simulink model "TCMSSystem"  (R2019b)
settings: configuration reference "ConfigSet_TCMSSystem_Reference" (kept outside this file)
model workspace (MAT data in the model file):
  Prm_TCMSSystem : Simulink.Parameter (value not decoded)
  SampleTime = 0.05
symbols that are objects in the model workspace (value not decoded): Prm_TCMSSystem
undefined symbols (not defined in the file): ADDIntervention, AK1Status, AK2Status, AKContactorStatus, AllDoorsClosed, AllLeftDoorsClosed, AllRightDoorsClosed, APS1Fault, APS1Isolated, APS1OutputVoltage, APS1Status, APS2Fault, APS2Isolated, APS2OutputVoltage, APS2Status, APSKAKContactor, ASCOEnd1, ASCOEnd2, ATBMode, ATCBypassMode, ATCStatusNotOK, ATOMode, ATPLowSpeedCutoutStatus, ATPMode, AuxCompressor, BatteryCurrent, BatteryIsolationContactor, BatteryTemperature, BatteryVoltage, BCG1Fault, BCG1Isolated, BCG1IsolationFailed, BCG1OutputCurrent, BCG1Status, BCG2Fault, BCG2Isolated, BCG2OutputCurrent, BCG2Status, BCGOutputVoltage, BECU1AxleLockedWheelSet1, BECU2AxleLockedWheelSet2, BECUFaulty, BECUMajorFault, BECUMinorFault, BECUStatus, BIC1Inside, BIC1Outside, BIC2Inside, BIC2Outside, Bogie, Bogie1WSPStatus, Bogie2WSPStatus, BogieFaulty, BogieIsolationStatus, BogieSupportedMass, BrakeCylinderPressureGauge, BrakeLoopCBTripped, BrakeLoopOpenTL, BrakeTrainLineStatus, BrakingDemand ... (+215)
libraries: TimersLib x257, simulink x137, LatchesLib x42, VectorOperationsLib x15, TestBenchLib x12, MathOperationsLib x2, FiltersLib x1
(part 5 of 16)

== system TCMSSystem/TCMSSystemPerVehicle/EnabledTCMSVehicle/TCMSDoors/DoorsDisplay/CabTrainDisplay ==
  TCMSConfig : Inport
  ElectricalSignals : Inport  Port=2
  AND : Logic  AllPortsSameDT=off  OutDataTypeStr=boolean
  Bus Selector : BusSelector  OutputSignals=CabActive
  Bus Selector1 : BusSelector  OutputSignals=HasCab
  CabActiveTrainDisplay : Subsystem  TreatAsAtomicUnit=on
  CabInactiveNoDisplay : Subsystem  TreatAsAtomicUnit=on
  Data Type Conversion : DataTypeConversion  OutDataTypeStr=uint32
  If : If
  Merge : Merge
  CabTrainDisplay : Outport
  wires:
  Merge/1 -> CabTrainDisplay/1
  CabInactiveNoDisplay/1(Out1) -> Merge/2
  CabActiveTrainDisplay/1(Out1) -> Merge/1
  If/2 -> CabInactiveNoDisplay/Action
  If/1 -> CabActiveTrainDisplay/Action
  Data Type Conversion/1 -> If/1
  AND/1 -> Data Type Conversion/1
  Bus Selector/1 -> AND/2  "<CabActive>"
  Bus Selector1/1 -> AND/1  "<HasCab>"
  TCMSConfig/1 -> Bus Selector1/1
  ElectricalSignals/1 -> Bus Selector/1, CabActiveTrainDisplay/1(ElectricalSignals)

== system TCMSSystem/TCMSSystemPerVehicle/EnabledTCMSVehicle/TCMSDoors/DoorsDisplay/TCMSVehicleInfo ==
  In Bus Element3 : Inport  PortName=DoorSystem  Element=Doors
  CommonVehicleConfig : Inport  Port=2
  In Bus Element : Inport  Port=3  PortName=ElectricalSignals  Element=DCUPower
  In Bus Element2 : Inport  Port=4  PortName=InputControlStates
  DoorsStatus1 : Subsystem
  OR : Logic  Operator=OR  Inputs=1  AllPortsSameDT=off  OutDataTypeStr=boolean
  Subsystem1 : Subsystem
  TCMSVehicleInfo : Outport
  UnexpectedDoorOpened : Outport  Port=2
  wires:
  In Bus Element3/1 -> DoorsStatus1/1(Doors)  "Doors"
  Subsystem1/1(TCMSDoorStatus) -> TCMSVehicleInfo/1
  CommonVehicleConfig/1 -> Subsystem1/1(CommonVehicleConfig)
  DoorsStatus1/1(DoorOpenStatus) -> Subsystem1/2(DoorOpenStatus)
  DoorsStatus1/16(DLSLFailure) -> Subsystem1/17(DLSLFailure)
  DoorsStatus1/17(DoorMajorFault) -> Subsystem1/18(DoorMajorFault)
  DoorsStatus1/12(DCUFailure) -> Subsystem1/13(DCUFailure)
  DoorsStatus1/3(DoorIsolatedStatus) -> Subsystem1/4(DoorIsolatedStatus)
  DoorsStatus1/15(DLSRFailure) -> Subsystem1/16(DLSRFailure)
  DoorsStatus1/13(DCSRFailure) -> Subsystem1/14(DCSRFailure)
  DoorsStatus1/14(DCSLFailure) -> Subsystem1/15(DCSLFailure)
  DoorsStatus1/10(DoorFailedToUnlock) -> Subsystem1/11(DoorFailedToUnlock)
  DoorsStatus1/4(DoorFaultStatus) -> Subsystem1/5(DoorFaultStatus)
  DoorsStatus1/7(DoorOpenObstruction) -> Subsystem1/8(DoorOpenObstruction)
  DoorsStatus1/8(DoorMotorCircuitFailure) -> Subsystem1/9(DoorMotorCircuitFailure)
  DoorsStatus1/2(DoorEmergencyReleasedStatus) -> Subsystem1/3(DoorEmergencyReleasedStatus)
  DoorsStatus1/6(DoorCloseObstruction) -> Subsystem1/7(DoorCloseObstruction)
  DoorsStatus1/5(DoorLockedStatus) -> Subsystem1/6(DoorLockedStatus)
  DoorsStatus1/11(DoorUnexpectedUnlocking) -> Subsystem1/12(DoorUnexpectedUnlocking)
  DoorsStatus1/9(DoorFailedToLock) -> Subsystem1/10(DoorFailedToLock)
  DoorsStatus1/18(UnexpectedDoorOpeningDetectedByCC) -> OR/1, Subsystem1/19(UnexpectedDoorOpeningDetectedByCC)
  OR/1 -> UnexpectedDoorOpened/1
  In Bus Element/1 -> Subsystem1/20(DCUPower)
  In Bus Element2/1 -> Subsystem1/21(InputControlStates)

== system TCMSSystem/TCMSSystemPerVehicle/EnabledTCMSVehicle/TCMSElectrical/ElectricalControl/Automatic Start Mode ==
  Key_Switch : Inport
  MS : Inport  Port=2
  TBC : Inport  Port=3
  WakeUp : Inport  Port=4
  Compare To Constant : simulink/Logic and Bit Operations/Compare To Constant  relop===  const=0  OutDataTypeStr=boolean
  Compare To Constant1 : simulink/Logic and Bit Operations/Compare To Constant  relop===  const=0  OutDataTypeStr=boolean
  Compare To Constant2 : simulink/Logic and Bit Operations/Compare To Constant  relop===  const=-100  OutDataTypeStr=boolean
  Logical Operator : Logic  Inputs=4  AllPortsSameDT=off  OutDataTypeStr=boolean
  TimerOnDelay NoInit : TimersLib/TimerOnDelay NoInit  UpperSaturationLimit=40  OutputTime=off  SampleTime=-1
      settings: SourceProductName=Sydac Utilities
  AutoStart : Outport
  wires:
  Key_Switch/1 -> Compare To Constant/1
  Compare To Constant/1 -> Logical Operator/1
  MS/1 -> Compare To Constant1/1
  Compare To Constant1/1 -> Logical Operator/2
  TBC/1 -> Compare To Constant2/1
  Compare To Constant2/1 -> Logical Operator/3
  WakeUp/1 -> TimerOnDelay NoInit/1
  Logical Operator/1 -> AutoStart/1
  TimerOnDelay NoInit/1 -> Logical Operator/4

== system TCMSSystem/TCMSSystemPerVehicle/EnabledTCMSVehicle/TCMSElectrical/ElectricalControl/Compressor_Start_Stop ==
  In Bus Element134 : Inport  PortName=PneumaticsSignals  Element=MainReservoirPressureGauge
  ActiveCab : Inport  Port=2
  NonActiveCab : Inport  Port=3
  AND19 : Logic  AllPortsSameDT=off  OutDataTypeStr=boolean
  AND20 : Logic  AllPortsSameDT=off  OutDataTypeStr=boolean
  AND21 : Logic  Operator=OR  AllPortsSameDT=off  OutDataTypeStr=boolean
  Compressor at DM1 : LatchesLib/SR Latch - Reset Priority  initial_condition=0
      settings: SourceProductName=Latches
  Compressor at DM2 : LatchesLib/SR Latch - Reset Priority  initial_condition=0
      settings: SourceProductName=Latches
  Constant3 : Constant  Value=800000
  Constant4 : Constant  Value=750000
  Constant5 : Constant  Value=1000000
  Data Type Conversion : DataTypeConversion
  Relational Operator : RelationalOperator  Operator=<=  OutDataTypeStr=boolean  RndMeth=Simplest
  Relational Operator1 : RelationalOperator  Operator=<=  OutDataTypeStr=boolean  RndMeth=Simplest
  Relational Operator2 : RelationalOperator  OutDataTypeStr=boolean  RndMeth=Simplest
  CompressorCmd : Outport
  wires:
  Relational Operator2/1 -> Compressor at DM2/2, Compressor at DM1/2
  Relational Operator/1 -> AND19/1
  Relational Operator1/1 -> AND20/1
  In Bus Element134/1 -> Relational Operator/1, Relational Operator1/1, Relational Operator2/1
  AND21/1 -> Data Type Conversion/1
  ActiveCab/1 -> AND19/2
  Compressor at DM1/1 -> AND21/1
  Constant4/1 -> Relational Operator1/2
  Compressor at DM2/1 -> AND21/2
  NonActiveCab/1 -> AND20/2
  Constant5/1 -> Relational Operator2/2
  AND19/1 -> Compressor at DM1/1
  AND20/1 -> Compressor at DM2/1
  Constant3/1 -> Relational Operator/2
  Data Type Conversion/1 -> CompressorCmd/1

== system TCMSSystem/TCMSSystemPerVehicle/EnabledTCMSVehicle/TCMSElectrical/ElectricalControl/Doors ==
  BusIn : Inport
  AllLeftDoorsClosed : Inport  Port=2
  Unused : Inport  Port=3
  AllRightDoorsClosed : Inport  Port=4
  AutoMode : Inport  Port=5
  In Bus Element : Inport  Port=6  PortName=ElectricalSignals  Element=LeftDoorEnable
  In Bus Element1 : Inport  Port=6  PortName=ElectricalSignals  Element=RightDoorEnable
  In Bus Element4 : Inport  Port=6  PortName=ElectricalSignals  Element=LeftHoldDoorClose
  In Bus Element5 : Inport  Port=6  PortName=ElectricalSignals  Element=RightHoldDoorClose
  In Bus Element2 : Inport  Port=7  PortName=CBTC  Element=LeftDoorCloseIndicator
  In Bus Element3 : Inport  Port=7  PortName=CBTC  Element=RightDoorCloseIndicator
  Bus Assignment3 : BusAssignment  AssignedSignals=LeftDoorAuth_Closed,LeftDoorAuth_Opened,RightDoorAuth_Closed,RightDoorAuth_Opened,RightDoorAuth_Opened_Op2_5,LeftDoorAuth_Opened_Op2_5,LeftDoorAuth_OpenedOP1,RightDoorAuth_OpenedOP1
  Constant : Constant  Value=0
  Constant1 : Constant  Value=0
  Data Type Conversion{3,12,17..18} (4 alike) : DataTypeConversion
  Demux4 : Demux  Outputs=16
  Mux7 : Mux  Inputs=8
  Mux8 : Mux  Inputs=8
  OR5 : Logic  Inputs=1  AllPortsSameDT=off  OutDataTypeStr=boolean
  OR6 : Logic  Inputs=1  AllPortsSameDT=off  OutDataTypeStr=boolean
  Subsystem4 : Subsystem
  Subsystem5 : Subsystem
  Subsystem6 : Subsystem
  Switch{,1..3} (4 alike) : Switch  Criteria=u2 > Threshold
  Terminator : Terminator
  Terminator1 : Terminator
  BusOut : Outport
  wires:
  Switch/1 -> Bus Assignment3/6
  Switch1/1 -> Bus Assignment3/7
  Data Type Conversion17/1 -> Bus Assignment3/4
  Subsystem6/1(RightDoorsAuth&Closed) -> Data Type Conversion17/1
  Data Type Conversion3/1 -> Bus Assignment3/2
  Data Type Conversion18/1 -> Bus Assignment3/5, [RDAO]
  Data Type Conversion12/1 -> Bus Assignment3/3, [LDAO]
  Bus Assignment3/1 -> BusOut/1
  Subsystem6/2(RightDoorsAuth&Opened) -> Data Type Conversion18/1
  Mux7/1 -> OR5/1
  OR5/1 -> Terminator/1  "LeftDoorsAuthorized"
  [RDAO] -> Switch3/1, Switch/3
  BusIn/1 -> Bus Assignment3/1
  Constant/1 -> Switch/1, Switch1/1
  Mux8/1 -> OR6/1
  Subsystem4/1(LeftDoorsAuth&Closed) -> Data Type Conversion3/1
  Subsystem4/2(LeftDoorsAuth&Opened) -> Data Type Conversion12/1
  Subsystem5/1(DoorAuthorized) -> Demux4/1
  [LDAO] -> Switch2/1, Switch1/3
  AllRightDoorsClosed/1 -> Subsystem6/2(AllRightDoorsClosed)
  OR6/1 -> Terminator1/1  "RightDoorsAuthorized"
  Unused/1 -> Subsystem5/1(In1)
  AllLeftDoorsClosed/1 -> Subsystem4/2(AllLeftDoorsClosed)
  Demux4/9 -> Mux8/1
  Demux4/10 -> Mux8/2
  Demux4/11 -> Mux8/3
  Demux4/12 -> Mux8/4
  Demux4/13 -> Mux8/5
  Demux4/14 -> Mux8/6
  Demux4/15 -> Mux8/7
  Demux4/16 -> Mux8/8
  Demux4/1 -> Mux7/1
  Demux4/2 -> Mux7/2
  Demux4/3 -> Mux7/3
  Demux4/4 -> Mux7/4
  Demux4/5 -> Mux7/5
  Demux4/6 -> Mux7/6
  Demux4/7 -> Mux7/7
  Demux4/8 -> Mux7/8
  In Bus Element/1 -> Subsystem4/1(LeftDoorsEnable)
  In Bus Element1/1 -> Subsystem6/1(RightDoorsEnable)
  In Bus Element2/1 -> Subsystem4/3(ATCLeftDoorCloseAuth)
  In Bus Element3/1 -> Subsystem6/3(ATCRightDoorCloseAuth)
  In Bus Element5/1 -> Subsystem6/4(RightHoldDooorClose)
  In Bus Element4/1 -> Subsystem4/4(LeftHoldDooorClose)
  Constant1/1 -> Switch2/3, Switch3/3
  AutoMode/1 -> Switch/2, Switch3/2, Switch2/2, Switch1/2
  Switch2/1 -> Bus Assignment3/8
  Switch3/1 -> Bus Assignment3/9

== system TCMSSystem/TCMSSystemPerVehicle/EnabledTCMSVehicle/TCMSElectrical/ElectricalControl/Subsystem ==
  note: SH: VCBs are closed by pressing the VCBCPB, hence implemented in electrical system.
      | If there is any new requirement for TCMS to close the VCB (apart from at the end of neutral section) shall be implemented here.
  note: VCB Open command in Faults
  In Bus Element : Inport  PortName=WireStates  Element=TW_POFFPB
  In Bus Element12 : Inport  PortName=WireStates  Element=TW_TPOR
  In Bus Element7 : Inport  Port=2  PortName=Environment  Element=NeutralSection
  In Bus Element1 : Inport  Port=2  PortName=Environment  Element=DamagedOHE
  In Bus Element9 : Inport  Port=2  PortName=Environment  Element=VehiclesPassedNS
  Fault : Inport  Port=3
  In Bus Element2 : Inport  Port=4  PortName=PantographSystem  Element=PantographPosition
  In Bus Element5 : Inport  Port=5  PortName=DisplayControl  Element=TCMSVCBOpenReq
  In Bus Element6 : Inport  Port=5  PortName=DisplayControl  Element=TCMSVCBCloseReq
  In Bus Element3 : Inport  Port=5  PortName=DisplayControl  Element=TCMSVCBResetReq
  In Bus Element8 : Inport  Port=5  PortName=DisplayControl  Element=TCMSReqCtrlVCBNS
  In Bus Element10 : Inport  Port=6  PortName=VCBState
  AND : Logic  AllPortsSameDT=off  OutDataTypeStr=boolean
  AND1 : Logic  AllPortsSameDT=off  OutDataTypeStr=boolean
  Chart : Stateflow chart  BlockKeywords=__PRM__SERIALIZED__DATA__:Stateflow Chart,Stateflow Diagram  TreatAsAtomicUnit=on
  Compare To Constant : simulink/Logic and Bit Operations/Compare To Constant  relop=>=  const=1  OutDataTypeStr=boolean
  Compare To Constant1 : simulink/Logic and Bit Operations/Compare To Constant  relop===  const=1  OutDataTypeStr=boolean
  Data Type Conversion : DataTypeConversion
  Logical Operator1 : Logic  Operator=OR  AllPortsSameDT=off  OutDataTypeStr=boolean
  Logical Operator2 : Logic  Operator=OR  Inputs=3  AllPortsSameDT=off  OutDataTypeStr=boolean
  Logical Operator3 : Logic  AllPortsSameDT=off  OutDataTypeStr=boolean
  Logical Operator4 : Logic  Operator=OR  AllPortsSameDT=off  OutDataTypeStr=boolean
  Logical Operator6 : Logic  Operator=OR  AllPortsSameDT=off  OutDataTypeStr=boolean
  MinimumDurationTimer : TimersLib/MinimumDurationTimer  UpperSaturationLimit=2  SampleTime=-1
      settings: SourceProductName=Sydac Utilities
  NOT : Logic  Operator=NOT  AllPortsSameDT=off  OutDataTypeStr=boolean
  Relational Operator : RelationalOperator  Operator=<  OutDataTypeStr=boolean  RndMeth=Simplest
  Unit Delay : UnitDelay  SampleTime=-1  HasFrameUpgradeWarning=on
  VCBC : Outport
  VCBO : Outport  Port=2
  BackupModeActive : Outport  Port=3
  TrainInNeutralSection : Outport  Port=4
  wires:
  Relational Operator/1 -> MinimumDurationTimer/1
  Logical Operator6/1 -> VCBO/1
  In Bus Element5/1 -> Logical Operator6/2
  Fault/1 -> Logical Operator3/2
  Compare To Constant/1 -> Data Type Conversion/1, Logical Operator3/1
  AND1/1 -> Logical Operator4/1, Unit Delay/1, Relational Operator/1
  In Bus Element1/1 -> Logical Operator4/2
  Logical Operator4/1 -> Logical Operator6/1
  Logical Operator1/1 -> VCBC/1
  MinimumDurationTimer/1 -> Logical Operator1/2
  Unit Delay/1 -> Relational Operator/2
  In Bus Element2/1 -> Compare To Constant1/1
  Compare To Constant1/1 -> Chart/4(PantographRaisedFully), AND/2  "PantographRaisedFully"
  AND/1 -> Logical Operator1/1
  In Bus Element6/1 -> Logical Operator2/2
  Logical Operator2/1 -> AND/1
  In Bus Element3/1 -> Logical Operator2/3
  NOT/1 -> AND1/2
  In Bus Element8/1 -> NOT/1
  In Bus Element7/1 -> AND1/1
  In Bus Element9/1 -> Compare To Constant/1
  Logical Operator3/1 -> BackupModeActive/1
  Data Type Conversion/1 -> TrainInNeutralSection/1
  In Bus Element12/1 -> Chart/1(TW_TPOR)
  Chart/1(VCBCloseReq) -> Logical Operator2/1
  In Bus Element/1 -> Chart/2(TW_POFF)
  In Bus Element10/1 -> Chart/3(VCBState)

== system TCMSSystem/TCMSSystemPerVehicle/EnabledTCMSVehicle/TCMSElectrical/ElectricalControl/Subsystem1 ==
  NonActiveCab : Inport
  HasCab : Inport  Port=2
  Mode : Inport  Port=3
  ActiveCab : Inport  Port=4
  TW_ReverseDirection : Inport  Port=5
  AND1 : Logic  Operator=OR  AllPortsSameDT=off  OutDataTypeStr=boolean
  AND{2,5..6,9} (4 alike) : Logic  AllPortsSameDT=off  OutDataTypeStr=boolean
  AND3 : Logic  Inputs=3  AllPortsSameDT=off  OutDataTypeStr=boolean
  ATO : simulink/Logic and Bit Operations/Compare To Constant  relop===  const=6  OutDataTypeStr=boolean
  ATP : simulink/Logic and Bit Operations/Compare To Constant  relop===  const=1  OutDataTypeStr=boolean
  NotInOFF : simulink/Logic and Bit Operations/Compare To Constant  relop=~=  const=0  OutDataTypeStr=boolean
  NotInStandby : simulink/Logic and Bit Operations/Compare To Constant  relop=~=  const=2  OutDataTypeStr=boolean
  RMF : simulink/Logic and Bit Operations/Compare To Constant  relop===  const=4  OutDataTypeStr=boolean
  RMR : simulink/Logic and Bit Operations/Compare To Constant  relop===  const=3  OutDataTypeStr=boolean
  Switch2 : Switch  Criteria=u2 > Threshold
  XOR : Logic  Operator=XOR  AllPortsSameDT=off  OutDataTypeStr=boolean
  ATPMode : Outport
  DrivingDirection : Outport  Port=2
  RMMode : Outport  Port=3
  AutoMode : Outport  Port=4
  wires:
  Mode/1 -> ATP/1, NotInOFF/1, NotInStandby/1, ATO/1, RMF/1, RMR/1
  HasCab/1 -> AND9/2, AND2/1
  XOR/1 -> RMMode/1  "RM"
  Switch2/1 -> DrivingDirection/1
  ActiveCab/1 -> AND3/2, AND6/2, AND5/2  "ActiveCabForward"
  AND5/1 -> XOR/1
  NonActiveCab/1 -> Switch2/1  "LastCabForward"
  RMF/1 -> AND6/1
  AND6/1 -> XOR/2
  ATP/1 -> AND9/1, AND1/1
  RMR/1 -> AND5/1
  AND9/1 -> ATPMode/1
  ATO/1 -> AND1/2
  AND2/1 -> AutoMode/1
  AND1/1 -> AND2/2
  TW_ReverseDirection/1 -> Switch2/2
  NotInOFF/1 -> AND3/1
  NotInStandby/1 -> AND3/3
  AND3/1 -> Switch2/3  "ActiveCabForward"

== system TCMSSystem/TCMSSystemPerVehicle/EnabledTCMSVehicle/TCMSElectrical/ElectricalControl/Subsystem10 ==
  Fault : Inport
  Cond : Inport  Port=2
  HasVCB : Inport  Port=3
  Reset : Inport  Port=4
  Data Type Conversion : DataTypeConversion
  Logical Operator1 : Logic  Inputs=3  AllPortsSameDT=off  OutDataTypeStr=boolean
  SR Latch - Reset Priority : LatchesLib/SR Latch - Reset Priority  initial_condition=0
      settings: SourceProductName=Latches
  Trig : Outport
  wires:
  Data Type Conversion/1 -> Trig/1
  SR Latch - Reset Priority/1 -> Data Type Conversion/1
  Logical Operator1/1 -> SR Latch - Reset Priority/1
  Fault/1 -> Logical Operator1/1
  Cond/1 -> Logical Operator1/2
  Reset/1 -> SR Latch - Reset Priority/2
  HasVCB/1 -> Logical Operator1/3

== system TCMSSystem/TCMSSystemPerVehicle/EnabledTCMSVehicle/TCMSElectrical/ElectricalControl/Subsystem11 ==
  Fault : Inport
  Cond : Inport  Port=2
  Cond1 : Inport  Port=3
  Data Type Conversion : DataTypeConversion
  Detect Decrease : simulink/Logic and Bit Operations/Detect Decrease  vinit=0.0  OutDataTypeStr=boolean
  Logical Operator1 : Logic  AllPortsSameDT=off  OutDataTypeStr=boolean
  Logical Operator2 : Logic  Operator=OR  AllPortsSameDT=off  OutDataTypeStr=boolean
  SR Latch - Reset Priority : LatchesLib/SR Latch - Reset Priority  initial_condition=0
      settings: SourceProductName=Latches
  Trig : Outport
  wires:
  Data Type Conversion/1 -> Trig/1
  Detect Decrease/1 -> Logical Operator2/1
  SR Latch - Reset Priority/1 -> Data Type Conversion/1
  Logical Operator1/1 -> SR Latch - Reset Priority/1
  Fault/1 -> Logical Operator1/1, Detect Decrease/1
  Cond/1 -> Logical Operator1/2
  Logical Operator2/1 -> SR Latch - Reset Priority/2
  Cond1/1 -> Logical Operator2/2

== system TCMSSystem/TCMSSystemPerVehicle/EnabledTCMSVehicle/TCMSElectrical/ElectricalControl/Subsystem12 ==
  Fault : Inport
  Cond : Inport  Port=2
  Cond1 : Inport  Port=3
  Data Type Conversion : DataTypeConversion
  Detect Decrease : simulink/Logic and Bit Operations/Detect Decrease  vinit=0.0  OutDataTypeStr=boolean
  Logical Operator1 : Logic  AllPortsSameDT=off  OutDataTypeStr=boolean
  Logical Operator2 : Logic  Operator=OR  AllPortsSameDT=off  OutDataTypeStr=boolean
  SR Latch - Reset Priority : LatchesLib/SR Latch - Reset Priority  initial_condition=0
      settings: SourceProductName=Latches
  Trig : Outport
  wires:
  Cond/1 -> Logical Operator1/2
  Fault/1 -> Detect Decrease/1, Logical Operator1/1
  Logical Operator1/1 -> SR Latch - Reset Priority/1
  SR Latch - Reset Priority/1 -> Data Type Conversion/1
  Detect Decrease/1 -> Logical Operator2/1
  Data Type Conversion/1 -> Trig/1
  Logical Operator2/1 -> SR Latch - Reset Priority/2
  Cond1/1 -> Logical Operator2/2

== system TCMSSystem/TCMSSystemPerVehicle/EnabledTCMSVehicle/TCMSElectrical/ElectricalControl/Subsystem13 ==
  Fault : Inport
  Cond : Inport  Port=2
  Cond1 : Inport  Port=3
  Data Type Conversion : DataTypeConversion
  Detect Decrease : simulink/Logic and Bit Operations/Detect Decrease  vinit=0.0  OutDataTypeStr=boolean
  Logical Operator1 : Logic  AllPortsSameDT=off  OutDataTypeStr=boolean
  Logical Operator2 : Logic  Operator=OR  AllPortsSameDT=off  OutDataTypeStr=boolean
  SR Latch - Reset Priority : LatchesLib/SR Latch - Reset Priority  initial_condition=0
      settings: SourceProductName=Latches
  Trig : Outport
  wires:
  Cond/1 -> Logical Operator1/2
  Fault/1 -> Detect Decrease/1, Logical Operator1/1
  Logical Operator1/1 -> SR Latch - Reset Priority/1
  SR Latch - Reset Priority/1 -> Data Type Conversion/1
  Detect Decrease/1 -> Logical Operator2/1
  Data Type Conversion/1 -> Trig/1
  Cond1/1 -> Logical Operator2/2
  Logical Operator2/1 -> SR Latch - Reset Priority/2

== system TCMSSystem/TCMSSystemPerVehicle/EnabledTCMSVehicle/TCMSElectrical/ElectricalControl/Subsystem14 ==
  Fault : Inport
  Cond : Inport  Port=2
  Cond1 : Inport  Port=3
  Data Type Conversion : DataTypeConversion
  Detect Decrease : simulink/Logic and Bit Operations/Detect Decrease  vinit=0.0  OutDataTypeStr=boolean
  Logical Operator1 : Logic  AllPortsSameDT=off  OutDataTypeStr=boolean
  Logical Operator2 : Logic  Operator=OR  AllPortsSameDT=off  OutDataTypeStr=boolean
  SR Latch - Reset Priority : LatchesLib/SR Latch - Reset Priority  initial_condition=0
      settings: SourceProductName=Latches
  Trig : Outport
  wires:
  Data Type Conversion/1 -> Trig/1
  Detect Decrease/1 -> Logical Operator2/1
  SR Latch - Reset Priority/1 -> Data Type Conversion/1
  Logical Operator1/1 -> SR Latch - Reset Priority/1
  Fault/1 -> Logical Operator1/1, Detect Decrease/1
  Cond/1 -> Logical Operator1/2
  Cond1/1 -> Logical Operator2/2
  Logical Operator2/1 -> SR Latch - Reset Priority/2

== system TCMSSystem/TCMSSystemPerVehicle/EnabledTCMSVehicle/TCMSElectrical/ElectricalControl/Subsystem15 ==
  Fault : Inport
  Cond : Inport  Port=2
  Data Type Conversion : DataTypeConversion
  Detect Decrease : simulink/Logic and Bit Operations/Detect Decrease  vinit=0.0  OutDataTypeStr=boolean
  Logical Operator1 : Logic  AllPortsSameDT=off  OutDataTypeStr=boolean
  SR Latch - Reset Priority : LatchesLib/SR Latch - Reset Priority  initial_condition=0
      settings: SourceProductName=Latches
  Trig : Outport
  wires:
  Cond/1 -> Logical Operator1/2
  Fault/1 -> Detect Decrease/1, Logical Operator1/1
  Logical Operator1/1 -> SR Latch - Reset Priority/1
  SR Latch - Reset Priority/1 -> Data Type Conversion/1
  Detect Decrease/1 -> SR Latch - Reset Priority/2
  Data Type Conversion/1 -> Trig/1

== system TCMSSystem/TCMSSystemPerVehicle/EnabledTCMSVehicle/TCMSElectrical/ElectricalControl/Subsystem16 ==
  Fault : Inport
  Cond : Inport  Port=2
  Data Type Conversion : DataTypeConversion
  Detect Decrease : simulink/Logic and Bit Operations/Detect Decrease  vinit=0.0  OutDataTypeStr=boolean
  Logical Operator1 : Logic  AllPortsSameDT=off  OutDataTypeStr=boolean
  SR Latch - Reset Priority : LatchesLib/SR Latch - Reset Priority  initial_condition=0
      settings: SourceProductName=Latches
  Trig : Outport
  wires:
  Data Type Conversion/1 -> Trig/1
  Detect Decrease/1 -> SR Latch - Reset Priority/2
  SR Latch - Reset Priority/1 -> Data Type Conversion/1
  Logical Operator1/1 -> SR Latch - Reset Priority/1
  Fault/1 -> Logical Operator1/1, Detect Decrease/1
  Cond/1 -> Logical Operator1/2

== system TCMSSystem/TCMSSystemPerVehicle/EnabledTCMSVehicle/TCMSElectrical/ElectricalControl/Subsystem17 ==
  Fault : Inport
  Cond : Inport  Port=2
  Cond1 : Inport  Port=3
  Data Type Conversion : DataTypeConversion
  Detect Decrease : simulink/Logic and Bit Operations/Detect Decrease  vinit=0.0  OutDataTypeStr=boolean
  Logical Operator1 : Logic  AllPortsSameDT=off  OutDataTypeStr=boolean
  Logical Operator2 : Logic  Operator=OR  AllPortsSameDT=off  OutDataTypeStr=boolean
  SR Latch - Reset Priority : LatchesLib/SR Latch - Reset Priority  initial_condition=0
      settings: SourceProductName=Latches
  Trig : Outport
  wires:
  Cond/1 -> Logical Operator1/2
  Fault/1 -> Detect Decrease/1, Logical Operator1/1
  Logical Operator1/1 -> SR Latch - Reset Priority/1
  SR Latch - Reset Priority/1 -> Data Type Conversion/1
  Detect Decrease/1 -> Logical Operator2/1
  Data Type Conversion/1 -> Trig/1
  Logical Operator2/1 -> SR Latch - Reset Priority/2
  Cond1/1 -> Logical Operator2/2

== system TCMSSystem/TCMSSystemPerVehicle/EnabledTCMSVehicle/TCMSElectrical/ElectricalControl/Subsystem18 ==
  Fault : Inport
  Cond : Inport  Port=2
  Cond1 : Inport  Port=3
  Data Type Conversion : DataTypeConversion
  Detect Decrease : simulink/Logic and Bit Operations/Detect Decrease  vinit=0.0  OutDataTypeStr=boolean
  Logical Operator1 : Logic  AllPortsSameDT=off  OutDataTypeStr=boolean
  Logical Operator2 : Logic  Operator=OR  AllPortsSameDT=off  OutDataTypeStr=boolean
  SR Latch - Reset Priority : LatchesLib/SR Latch - Reset Priority  initial_condition=0
      settings: SourceProductName=Latches
  Trig : Outport
  wires:
  Data Type Conversion/1 -> Trig/1
  Detect Decrease/1 -> Logical Operator2/1
  SR Latch - Reset Priority/1 -> Data Type Conversion/1
  Logical Operator1/1 -> SR Latch - Reset Priority/1
  Fault/1 -> Logical Operator1/1, Detect Decrease/1
  Cond/1 -> Logical Operator1/2
  Cond1/1 -> Logical Operator2/2
  Logical Operator2/1 -> SR Latch - Reset Priority/2

== system TCMSSystem/TCMSSystemPerVehicle/EnabledTCMSVehicle/TCMSElectrical/ElectricalControl/Subsystem19 ==
  Open : Inport
  Close : Inport  Port=2
  Data Type Conversion : DataTypeConversion
  Logical Operator1 : Logic  AllPortsSameDT=off  OutDataTypeStr=boolean
  Logical Operator2 : Logic  Operator=NOT  AllPortsSameDT=off  OutDataTypeStr=boolean
  Trig : Outport
  wires:
  Open/1 -> Logical Operator1/1
  Close/1 -> Logical Operator2/1
  Logical Operator1/1 -> Data Type Conversion/1
  Logical Operator2/1 -> Logical Operator1/2
  Data Type Conversion/1 -> Trig/1

== system TCMSSystem/TCMSSystemPerVehicle/EnabledTCMSVehicle/TCMSElectrical/ElectricalControl/Subsystem2 ==
  TW_POFF : Inport
  TSDR_ON : Inport  Port=2
  KeySwitchStatus : Inport  Port=3
  ShutdownFailure : Inport  Port=4
  TW_ShutdownFailure : Inport  Port=5
  Logical Operator : Logic  Inputs=3  AllPortsSameDT=off  OutDataTypeStr=boolean
  Logical Operator1 : Logic  Operator=NOT  AllPortsSameDT=off  OutDataTypeStr=boolean
  Logical Operator2 : Logic  Operator=NOT  AllPortsSameDT=off  OutDataTypeStr=boolean
  Logical Operator3 : Logic  AllPortsSameDT=off  OutDataTypeStr=boolean
  Logical Operator4 : Logic  Operator=NOT  AllPortsSameDT=off  OutDataTypeStr=boolean
  TimerOnDelay NoInit : TimersLib/TimerOnDelay NoInit  UpperSaturationLimit=5  OutputTime=off  SampleTime=-1
      settings: SourceProductName=Sydac Utilities
  TSDDR : Outport
  TCMS_TSDR : Outport  Port=2
  wires:
  TW_POFF/1 -> Logical Operator/1
  TSDR_ON/1 -> Logical Operator3/1
  TimerOnDelay NoInit/1 -> TSDDR/1
  KeySwitchStatus/1 -> Logical Operator1/1
  Logical Operator1/1 -> Logical Operator/2
  Logical Operator/1 -> TCMS_TSDR/1
  ShutdownFailure/1 -> Logical Operator2/1
  Logical Operator2/1 -> Logical Operator/3
  Logical Operator3/1 -> TimerOnDelay NoInit/1
  TW_ShutdownFailure/1 -> Logical Operator4/1
  Logical Operator4/1 -> Logical Operator3/2

== system TCMSSystem/TCMSSystemPerVehicle/EnabledTCMSVehicle/TCMSElectrical/ElectricalControl/Subsystem20 ==
  Open : Inport
  Close : Inport  Port=2
  Data Type Conversion : DataTypeConversion
  Logical Operator1 : Logic  AllPortsSameDT=off  OutDataTypeStr=boolean
  Logical Operator2 : Logic  Operator=NOT  AllPortsSameDT=off  OutDataTypeStr=boolean
  Trig : Outport
  wires:
  Logical Operator2/1 -> Logical Operator1/2
  Logical Operator1/1 -> Data Type Conversion/1
  Close/1 -> Logical Operator2/1
  Open/1 -> Logical Operator1/1
  Data Type Conversion/1 -> Trig/1

== system TCMSSystem/TCMSSystemPerVehicle/EnabledTCMSVehicle/TCMSElectrical/ElectricalControl/Subsystem21 ==
  Open : Inport
  Close : Inport  Port=2
  Data Type Conversion : DataTypeConversion
  Logical Operator1 : Logic  AllPortsSameDT=off  OutDataTypeStr=boolean
  Logical Operator2 : Logic  Operator=NOT  AllPortsSameDT=off  OutDataTypeStr=boolean
  Trig : Outport
  wires:
  Open/1 -> Logical Operator1/1
  Close/1 -> Logical Operator2/1
  Logical Operator1/1 -> Data Type Conversion/1
  Logical Operator2/1 -> Logical Operator1/2
  Data Type Conversion/1 -> Trig/1

== system TCMSSystem/TCMSSystemPerVehicle/EnabledTCMSVehicle/TCMSElectrical/ElectricalControl/Subsystem22 ==
  Open : Inport
  Close : Inport  Port=2
  Data Type Conversion : DataTypeConversion
  Logical Operator1 : Logic  AllPortsSameDT=off  OutDataTypeStr=boolean
  Logical Operator2 : Logic  Operator=NOT  AllPortsSameDT=off  OutDataTypeStr=boolean
  Trig : Outport
  wires:
  Logical Operator2/1 -> Logical Operator1/2
  Logical Operator1/1 -> Data Type Conversion/1
  Close/1 -> Logical Operator2/1
  Open/1 -> Logical Operator1/1
  Data Type Conversion/1 -> Trig/1

== system TCMSSystem/TCMSSystemPerVehicle/EnabledTCMSVehicle/TCMSElectrical/ElectricalControl/Subsystem3 ==
  Fault : Inport
  LV : Inport  Port=2
  Data Type Conversion : DataTypeConversion
  Detect Decrease : simulink/Logic and Bit Operations/Detect Decrease  vinit=0.0  OutDataTypeStr=boolean
  Logical Operator1 : Logic  AllPortsSameDT=off  OutDataTypeStr=boolean
  SR Latch - Reset Priority : LatchesLib/SR Latch - Reset Priority  initial_condition=0
      settings: SourceProductName=Latches
  Trig : Outport
  wires:
  LV/1 -> Logical Operator1/2
  Fault/1 -> Detect Decrease/1, Logical Operator1/1
  Logical Operator1/1 -> SR Latch - Reset Priority/1
  SR Latch - Reset Priority/1 -> Data Type Conversion/1
  Detect Decrease/1 -> SR Latch - Reset Priority/2
  Data Type Conversion/1 -> Trig/1

== system TCMSSystem/TCMSSystemPerVehicle/EnabledTCMSVehicle/TCMSElectrical/ElectricalControl/Subsystem4 ==
  Fault : Inport
  LV : Inport  Port=2
  Data Type Conversion : DataTypeConversion
  Detect Decrease : simulink/Logic and Bit Operations/Detect Decrease  vinit=0.0  OutDataTypeStr=boolean
  Logical Operator1 : Logic  AllPortsSameDT=off  OutDataTypeStr=boolean
  SR Latch - Reset Priority : LatchesLib/SR Latch - Reset Priority  initial_condition=0
      settings: SourceProductName=Latches
  Trig : Outport
  wires:
  Data Type Conversion/1 -> Trig/1
  Detect Decrease/1 -> SR Latch - Reset Priority/2
  SR Latch - Reset Priority/1 -> Data Type Conversion/1
  Logical Operator1/1 -> SR Latch - Reset Priority/1
  Fault/1 -> Logical Operator1/1, Detect Decrease/1
  LV/1 -> Logical Operator1/2

== system TCMSSystem/TCMSSystemPerVehicle/EnabledTCMSVehicle/TCMSElectrical/ElectricalControl/Subsystem5 ==
  Fault : Inport
  VCB : Inport  Port=2
  Data Type Conversion : DataTypeConversion
  Detect Decrease : simulink/Logic and Bit Operations/Detect Decrease  vinit=0.0  OutDataTypeStr=boolean
  Logical Operator1 : Logic  AllPortsSameDT=off  OutDataTypeStr=boolean
  SR Latch - Reset Priority : LatchesLib/SR Latch - Reset Priority  initial_condition=0
      settings: SourceProductName=Latches
  Trig : Outport
  wires:
  VCB/1 -> Logical Operator1/2
  Fault/1 -> Detect Decrease/1, Logical Operator1/1
  Logical Operator1/1 -> SR Latch - Reset Priority/1
  SR Latch - Reset Priority/1 -> Data Type Conversion/1
  Detect Decrease/1 -> SR Latch - Reset Priority/2
  Data Type Conversion/1 -> Trig/1

== system TCMSSystem/TCMSSystemPerVehicle/EnabledTCMSVehicle/TCMSElectrical/ElectricalControl/Subsystem6 ==
  Fault : Inport
  VCB : Inport  Port=2
  Data Type Conversion : DataTypeConversion
  Detect Decrease : simulink/Logic and Bit Operations/Detect Decrease  vinit=0.0  OutDataTypeStr=boolean
  Logical Operator1 : Logic  AllPortsSameDT=off  OutDataTypeStr=boolean
  SR Latch - Reset Priority : LatchesLib/SR Latch - Reset Priority  initial_condition=0
      settings: SourceProductName=Latches
  Trig : Outport
  wires:
  Data Type Conversion/1 -> Trig/1
  Detect Decrease/1 -> SR Latch - Reset Priority/2
  SR Latch - Reset Priority/1 -> Data Type Conversion/1
  Logical Operator1/1 -> SR Latch - Reset Priority/1
  Fault/1 -> Logical Operator1/1, Detect Decrease/1
  VCB/1 -> Logical Operator1/2

== system TCMSSystem/TCMSSystemPerVehicle/EnabledTCMSVehicle/TCMSElectrical/ElectricalControl/Subsystem7 ==
  Fault : Inport
  VCB : Inport  Port=2
  Data Type Conversion : DataTypeConversion
  Detect Decrease : simulink/Logic and Bit Operations/Detect Decrease  vinit=0.0  OutDataTypeStr=boolean
  Logical Operator1 : Logic  AllPortsSameDT=off  OutDataTypeStr=boolean
  SR Latch - Reset Priority : LatchesLib/SR Latch - Reset Priority  initial_condition=0
      settings: SourceProductName=Latches
  Trig : Outport
  wires:
  VCB/1 -> Logical Operator1/2
  Fault/1 -> Detect Decrease/1, Logical Operator1/1
  Logical Operator1/1 -> SR Latch - Reset Priority/1
  SR Latch - Reset Priority/1 -> Data Type Conversion/1
  Detect Decrease/1 -> SR Latch - Reset Priority/2
  Data Type Conversion/1 -> Trig/1

== system TCMSSystem/TCMSSystemPerVehicle/EnabledTCMSVehicle/TCMSElectrical/ElectricalControl/Subsystem8 ==
  Fault : Inport
  VCB : Inport  Port=2
  Data Type Conversion : DataTypeConversion
  Detect Decrease : simulink/Logic and Bit Operations/Detect Decrease  vinit=0.0  OutDataTypeStr=boolean
  Logical Operator1 : Logic  AllPortsSameDT=off  OutDataTypeStr=boolean
  SR Latch - Reset Priority : LatchesLib/SR Latch - Reset Priority  initial_condition=0
      settings: SourceProductName=Latches
  Trig : Outport
  wires:
  Data Type Conversion/1 -> Trig/1
  Detect Decrease/1 -> SR Latch - Reset Priority/2
  SR Latch - Reset Priority/1 -> Data Type Conversion/1
  Logical Operator1/1 -> SR Latch - Reset Priority/1
  Fault/1 -> Logical Operator1/1, Detect Decrease/1
  VCB/1 -> Logical Operator1/2

== system TCMSSystem/TCMSSystemPerVehicle/EnabledTCMSVehicle/TCMSElectrical/ElectricalControl/Subsystem9 ==
  Fault : Inport
  Cond : Inport  Port=2
  Data Type Conversion : DataTypeConversion
  Detect Decrease : simulink/Logic and Bit Operations/Detect Decrease  vinit=0.0  OutDataTypeStr=boolean
  Logical Operator1 : Logic  AllPortsSameDT=off  OutDataTypeStr=boolean
  SR Latch - Reset Priority : LatchesLib/SR Latch - Reset Priority  initial_condition=0
      settings: SourceProductName=Latches
  Trig : Outport
  wires:
  Cond/1 -> Logical Operator1/2
  Fault/1 -> Detect Decrease/1, Logical Operator1/1
  Logical Operator1/1 -> SR Latch - Reset Priority/1
  SR Latch - Reset Priority/1 -> Data Type Conversion/1
  Detect Decrease/1 -> SR Latch - Reset Priority/2
  Data Type Conversion/1 -> Trig/1

== system TCMSSystem/TCMSSystemPerVehicle/EnabledTCMSVehicle/TCMSElectrical/ElectricalDisplay/APSScreen ==
  note: BatteryScreen
  BusIn : Inport
  In Bus Element8 : Inport  Port=2  PortName=ElectricalSignals  Element=APS1Status
  In Bus Element9 : Inport  Port=2  PortName=ElectricalSignals  Element=APS2Status
  In Bus Element27 : Inport  Port=2  PortName=ElectricalSignals  Element=APS1Fault
  In Bus Element28 : Inport  Port=2  PortName=ElectricalSignals  Element=APS2Fault
  In Bus Element29 : Inport  Port=2  PortName=ElectricalSignals  Element=APS1Isolated
  In Bus Element30 : Inport  Port=2  PortName=ElectricalSignals  Element=APS2Isolated
  In Bus Element31 : Inport  Port=2  PortName=ElectricalSignals  Element=APS1OutputVoltage
  In Bus Element32 : Inport  Port=2  PortName=ElectricalSignals  Element=APS2OutputVoltage
  In Bus Element33 : Inport  Port=2  PortName=ElectricalSignals  Element=AK1Status
  In Bus Element34 : Inport  Port=2  PortName=ElectricalSignals  Element=AK2Status
  In Bus Element35 : Inport  Port=2  PortName=ElectricalSignals  Element=K1Status
  In Bus Element36 : Inport  Port=2  PortName=ElectricalSignals  Element=K2Status
  In Bus Element1 : Inport  Port=2  PortName=ElectricalSignals  Element=APSCBTripped
  Bus Assignment2 : BusAssignment  AssignedSignals=APS1Status,APS2Status,AK1Status,K1Status,AK2Status,K2Status,APS1Isolated,APS2Isolated,APS1OutputVoltage,APS2OutputVoltage,APS1Fault,APS2Fault
  Data Type Conversion{2,8..11,21..22,25..27} (10 alike) : DataTypeConversion
  Logical Operator : Logic  Operator=OR  AllPortsSameDT=off  OutDataTypeStr=boolean
  Logical Operator1 : Logic  Operator=OR  AllPortsSameDT=off  OutDataTypeStr=boolean
  BusOut : Outport
  wires:
  In Bus Element32/1 -> Bus Assignment2/11
  In Bus Element31/1 -> Bus Assignment2/10
  Bus Assignment2/1 -> BusOut/1
  Data Type Conversion9/1 -> Bus Assignment2/4
  In Bus Element30/1 -> Data Type Conversion2/1
  Data Type Conversion22/1 -> Bus Assignment2/6
  Data Type Conversion25/1 -> Bus Assignment2/12
  Data Type Conversion8/1 -> Bus Assignment2/5
  Data Type Conversion2/1 -> Bus Assignment2/9
  BusIn/1 -> Bus Assignment2/1
  In Bus Element28/1 -> Logical Operator/1
  Data Type Conversion27/1 -> Bus Assignment2/8
  Data Type Conversion26/1 -> Bus Assignment2/13
  In Bus Element34/1 -> Data Type Conversion22/1
  Data Type Conversion10/1 -> Bus Assignment2/2
  In Bus Element8/1 -> Data Type Conversion10/1
  In Bus Element9/1 -> Data Type Conversion11/1
  In Bus Element29/1 -> Data Type Conversion27/1
  In Bus Element35/1 -> Data Type Conversion8/1
  Data Type Conversion21/1 -> Bus Assignment2/7
  Data Type Conversion11/1 -> Bus Assignment2/3
  In Bus Element33/1 -> Data Type Conversion9/1
  In Bus Element27/1 -> Logical Operator1/1
  In Bus Element36/1 -> Data Type Conversion21/1
  In Bus Element1/1 -> Logical Operator/2, Logical Operator1/2
  Logical Operator1/1 -> Data Type Conversion25/1
  Logical Operator/1 -> Data Type Conversion26/1

== system TCMSSystem/TCMSSystemPerVehicle/EnabledTCMSVehicle/TCMSElectrical/ElectricalDisplay/BatteryScreen ==
  note: BatteryScreen
  BusIn : Inport
  In Bus Element4 : Inport  Port=2  PortName=ElectricalSignals  Element=BCG1Status
  In Bus Element5 : Inport  Port=2  PortName=ElectricalSignals  Element=BCG2Status
  In Bus Element6 : Inport  Port=2  PortName=ElectricalSignals  Element=BCGOutputVoltage
  In Bus Element7 : Inport  Port=2  PortName=ElectricalSignals  Element=BCG1OutputCurrent
  In Bus Element8 : Inport  Port=2  PortName=ElectricalSignals  Element=BCG2OutputCurrent
  In Bus Element : Inport  Port=2  PortName=ElectricalSignals  Element=BatteryVoltage
  In Bus Element1 : Inport  Port=2  PortName=ElectricalSignals  Element=BatteryCurrent
  In Bus Element2 : Inport  Port=2  PortName=ElectricalSignals  Element=BatteryTemperature
  In Bus Element3 : Inport  Port=2  PortName=ElectricalSignals  Element=BCG1Fault
  In Bus Element9 : Inport  Port=2  PortName=ElectricalSignals  Element=BCG2Fault
  In Bus Element11 : Inport  Port=2  PortName=ElectricalSignals  Element=BCG1Isolated
  In Bus Element12 : Inport  Port=2  PortName=ElectricalSignals  Element=BCG2Isolated
  In Bus Element10 : Inport  Port=2  PortName=ElectricalSignals  Element=BCG1IsolationFailed
  Add : Sum
  Bus Assignment2 : BusAssignment  AssignedSignals=BCG1Status,BCG2Status,BCG1Fault,BCG2Fault,BCGOutputVoltage,BCG1OutputCurrent,BCG2OutputCurrent,TotalOutputCurrent,BatteryVoltage,BatteryCurrent,BatteryTemperature,BCG1Isolated,BCG2Isolated,BCG1IsolationFailed
  Data Type Conversion1 : DataTypeConversion
  Data Type Conversion28 : DataTypeConversion
  BusOut : Outport
  wires:
  In Bus Element4/1 -> Data Type Conversion1/1
  Bus Assignment2/1 -> BusOut/1
  BusIn/1 -> Bus Assignment2/1
  In Bus Element5/1 -> Data Type Conversion28/1
  In Bus Element6/1 -> Bus Assignment2/6
  In Bus Element/1 -> Bus Assignment2/10
  In Bus Element1/1 -> Bus Assignment2/11
  In Bus Element2/1 -> Bus Assignment2/12
  Data Type Conversion28/1 -> Bus Assignment2/3
  Data Type Conversion1/1 -> Bus Assignment2/2
  In Bus Element7/1 -> Add/1, Bus Assignment2/7
  Add/1 -> Bus Assignment2/9
  In Bus Element8/1 -> Add/2, Bus Assignment2/8
  In Bus Element3/1 -> Bus Assignment2/4
  In Bus Element9/1 -> Bus Assignment2/5
  In Bus Element11/1 -> Bus Assignment2/13
  In Bus Element12/1 -> Bus Assignment2/14
  In Bus Element10/1 -> Bus Assignment2/15

== system TCMSSystem/TCMSSystemPerVehicle/EnabledTCMSVehicle/TCMSElectrical/ElectricalDisplay/BrakeLoopInterlock ==
  note: BrakeLoopInterlockScreen
  BusIn : Inport
  In Bus Element : Inport  Port=2  PortName=PantographSignals  Element=BrakeLoopADDIntervention
  In Bus Element2 : Inport  Port=3  PortName=ElectricalTrainWire  Element=BrakeLoopCBTripped
  Bus Assignment7 : BusAssignment  AssignedSignals=ADDIntervention,BrakeLoopCBTripped
  Data Type Conversion : DataTypeConversion
  Data Type Conversion1 : DataTypeConversion
  BusOut : Outport
  wires:
  Bus Assignment7/1 -> BusOut/1
  BusIn/1 -> Bus Assignment7/1
  In Bus Element/1 -> Data Type Conversion/1
  Data Type Conversion/1 -> Bus Assignment7/2
  In Bus Element2/1 -> Data Type Conversion1/1
  Data Type Conversion1/1 -> Bus Assignment7/3

== system TCMSSystem/TCMSSystemPerVehicle/EnabledTCMSVehicle/TCMSElectrical/ElectricalDisplay/BrakeScreen ==
  note: BatteryScreen
  BusIn : Inport
  In Bus Element18 : Inport  Port=2  PortName=ElectricalSignals  Element=BrakeTrainLine
  In Bus Element19 : Inport  Port=2  PortName=ElectricalSignals  Element=MotorTrainLine
  In Bus Element20 : Inport  Port=2  PortName=ElectricalSignals  Element=FSB1Line
  In Bus Element21 : Inport  Port=2  PortName=ElectricalSignals  Element=FSB2Line
  In Bus Element22 : Inport  Port=2  PortName=ElectricalSignals  Element=EB1Line
  In Bus Element23 : Inport  Port=2  PortName=ElectricalSignals  Element=EB2Line
  Bus Assignment2 : BusAssignment  AssignedSignals=BrakeTrainLineStatus,MotorTrainLineStatus,FSB1LineStatus,FSB2LineStatus,EB1LineStatus,EB2LineStatus
  Data Type Conversion{13,15..19} (6 alike) : DataTypeConversion
  BusOut : Outport
  wires:
  BusIn/1 -> Bus Assignment2/1
  Bus Assignment2/1 -> BusOut/1
  Data Type Conversion16/1 -> Bus Assignment2/4
  Data Type Conversion13/1 -> Bus Assignment2/2
  In Bus Element23/1 -> Data Type Conversion19/1
  Data Type Conversion18/1 -> Bus Assignment2/6
  In Bus Element19/1 -> Data Type Conversion15/1
  In Bus Element18/1 -> Data Type Conversion13/1
  In Bus Element21/1 -> Data Type Conversion17/1
  Data Type Conversion17/1 -> Bus Assignment2/5
  Data Type Conversion15/1 -> Bus Assignment2/3
  In Bus Element22/1 -> Data Type Conversion18/1
  Data Type Conversion19/1 -> Bus Assignment2/7
  In Bus Element20/1 -> Data Type Conversion16/1

== system TCMSSystem/TCMSSystemPerVehicle/EnabledTCMSVehicle/TCMSElectrical/ElectricalDisplay/EBLoopInterlockScreen ==
  note: EBLoopInterlockScreen
  BusIn : Inport
  In Bus Element : Inport  Port=2  PortName=ElectricalSignals  Element=EBbyNonCabEnabled
  In Bus Element1 : Inport  Port=2  PortName=ElectricalSignals  Element=EBbyMC
  In Bus Element2 : Inport  Port=2  PortName=ElectricalSignals  Element=EBbyBrakeLoop
  In Bus Element3 : Inport  Port=2  PortName=ElectricalSignals  Element=EBbyDeadMan
  In Bus Element4 : Inport  Port=2  PortName=ElectricalSignals  Element=EBApplied
  In Bus Element13 : Inport  Port=2  PortName=ElectricalSignals  Element=EBApplied
  In Bus Element11 : Inport  Port=2  PortName=ElectricalSignals  Element=CabActive
  In Bus Element7 : Inport  Port=2  PortName=ElectricalSignals  Element=CabActive
  In Bus Element8 : Inport  Port=2  PortName=ElectricalSignals  Element=EBbyCC
  In Bus Element9 : Inport  Port=2  PortName=ElectricalSignals  Element=EBdueToATCZeroSpeed
  In Bus Element6 : Inport  Port=2  PortName=ElectricalSignals  Element=EBbyPB
  In Bus Element10 : Inport  Port=2  PortName=ElectricalSignals  Element=ZeroSpeed
  In Bus Element5 : Inport  Port=3  PortName=InputControls  Element=ModeSelector
  In Bus Element12 : Inport  Port=4  PortName=TCMSSystemVehicleConfig  Element=IsFirstVehicle
  AND{1,3,5..8} (6 alike) : Logic  Inputs=3  AllPortsSameDT=off  OutDataTypeStr=boolean
  AND{10,12..14} (4 alike) : Logic  Operator=NOT  AllPortsSameDT=off  OutDataTypeStr=boolean
  AND{2,4,9,11} (4 alike) : Logic  AllPortsSameDT=off  OutDataTypeStr=boolean
  Bus Assignment7 : BusAssignment  AssignedSignals=EBForNonCabEnabled,EBForNonDirectionSelected,EBDueToPushButton,EBByMC,EBByBrakeLoop,EBDueToDeadman,EBByCC,EBDueToATCZeroSpeed
  Data Type Conversion{1..2,40,43..47} (8 alike) : DataTypeConversion
  OFF : simulink/Logic and Bit Operations/Compare To Constant  relop===  const=0  OutDataTypeStr=boolean
  OR : Logic  Operator=OR  AllPortsSameDT=off  OutDataTypeStr=boolean
  SR Latch - Reset Priority : LatchesLib/SR Latch - Reset Priority  initial_condition=0
      settings: SourceProductName=Latches
  SR Latch - Reset Priority1 : LatchesLib/SR Latch - Reset Priority  initial_condition=0
      settings: SourceProductName=Latches
  Standby : simulink/Logic and Bit Operations/Compare To Constant  relop===  const=2  OutDataTypeStr=boolean
  Terminator : Terminator
  BusOut : Outport
  wires:
  In Bus Element4/1 -> AND8/1, AND7/1, AND2/1, AND3/2, AND1/2, AND4/2, AND5/2, AND6/2
  Bus Assignment7/1 -> BusOut/1
  AND3/1 -> Data Type Conversion40/1
  AND1/1 -> Data Type Conversion46/1
  In Bus Element2/1 -> AND5/1
  AND6/1 -> Data Type Conversion45/1
  OFF/1 -> OR/1
  Data Type Conversion40/1 -> Bus Assignment7/2
  AND2/1 -> Data Type Conversion47/1
  In Bus Element5/1 -> OFF/1, Standby/1
  In Bus Element6/1 -> AND2/2
  AND5/1 -> Data Type Conversion44/1
  In Bus Element3/1 -> AND6/1
  In Bus Element1/1 -> AND4/1
  Standby/1 -> OR/2
  AND4/1 -> Data Type Conversion43/1
  OR/1 -> AND11/2
  BusIn/1 -> Bus Assignment7/1
  Data Type Conversion46/1 -> Bus Assignment7/3
  Data Type Conversion47/1 -> Bus Assignment7/4
  Data Type Conversion43/1 -> Bus Assignment7/5
  Data Type Conversion44/1 -> Bus Assignment7/6
  Data Type Conversion45/1 -> Bus Assignment7/7
  AND7/1 -> Data Type Conversion1/1
  In Bus Element8/1 -> AND7/2
  AND8/1 -> Data Type Conversion2/1
  In Bus Element9/1 -> AND8/2
  Data Type Conversion1/1 -> Bus Assignment7/8
  Data Type Conversion2/1 -> Bus Assignment7/9
  AND9/1 -> SR Latch - Reset Priority/1
  In Bus Element10/1 -> AND10/1
  AND10/1 -> AND11/1, AND9/1
  AND11/1 -> SR Latch - Reset Priority1/1
  SR Latch - Reset Priority/1 -> AND3/1
  SR Latch - Reset Priority1/1 -> AND1/1
  AND13/1 -> SR Latch - Reset Priority/2
  AND12/1 -> SR Latch - Reset Priority1/2
  In Bus Element/1 -> Terminator/1
  In Bus Element11/1 -> AND14/1
  AND14/1 -> AND9/2
  In Bus Element12/1 -> AND8/3, AND7/3, AND5/3, AND1/3, AND3/3
  In Bus Element7/1 -> AND6/3
  In Bus Element13/1 -> AND13/1, AND12/1

== system TCMSSystem/TCMSSystemPerVehicle/EnabledTCMSVehicle/TCMSElectrical/ElectricalDisplay/EnableToRunScreen ==
  note: EnableToRunScreen
  BusIn : Inport
  In Bus Element14 : Inport  Port=2  PortName=ElectricalSignals
  In Bus Element16 : Inport  Port=3  PortName=CBTC
  In Bus Element15 : Inport  Port=4  PortName=WireStates
  Bus Assignment7 : BusAssignment  AssignedSignals=HighVoltageMissing,CabNotEnabled,DrivingModeNotOK,TrainDirectionMissing,ATCStatusNotOK,TrainReadyNotOK,TooManyRPressureCutout,TooManyEPICCutout,TooManyBogieIsolated,ZVRDNotActive,MotoringTLDeenergized,BrakeLoopOpenTL,ParkingBrakeActiveTL,DoorLoopOpenTL
  Bus Selector : BusSelector  OutputSignals=NoLineVoltage,NoCabActive,NoModeSelected,NoDirectionSelected,ATCStatusNotOK,TrainReadyNotOK,TooManyRPRESS,TooManyEPIC,TooManyBogies,ZVRDNotActive,MotoringTLDeenergized,BrakeLoopCutout,ParkBrakeApplied,DoorLoopNotOK
  CabUnitDisplay : Subsystem
  BusOut : Outport
  wires:
  BusIn/1 -> Bus Assignment7/1
  Bus Assignment7/1 -> BusOut/1
  In Bus Element14/1 -> CabUnitDisplay/1(ElectricalSignals)
  In Bus Element15/1 -> CabUnitDisplay/2(WireStates)
  In Bus Element16/1 -> CabUnitDisplay/3(CBTC)
  CabUnitDisplay/1(CabUnitDisplay) -> Bus Selector/1  "CabUnitDisplay"
  Bus Selector/1 -> Bus Assignment7/2  "<NoLineVoltage>"
  Bus Selector/2 -> Bus Assignment7/3  "<NoCabActive>"
  Bus Selector/3 -> Bus Assignment7/4  "<NoModeSelected>"
  Bus Selector/4 -> Bus Assignment7/5  "<NoDirectionSelected>"
  Bus Selector/5 -> Bus Assignment7/6  "<ATCStatusNotOK>"
  Bus Selector/6 -> Bus Assignment7/7  "<TrainReadyNotOK>"
  Bus Selector/7 -> Bus Assignment7/8  "<TooManyRPRESS>"
  Bus Selector/8 -> Bus Assignment7/9  "<TooManyEPIC>"
  Bus Selector/9 -> Bus Assignment7/10  "<TooManyBogies>"
  Bus Selector/10 -> Bus Assignment7/11  "<ZVRDNotActive>"
  Bus Selector/11 -> Bus Assignment7/12  "<MotoringTLDeenergized>"
  Bus Selector/12 -> Bus Assignment7/13  "<BrakeLoopCutout>"
  Bus Selector/13 -> Bus Assignment7/14  "<ParkBrakeApplied>"
  Bus Selector/14 -> Bus Assignment7/15  "<DoorLoopNotOK>"
